simulink model "Assignment_4"  (R2023a)
settings: Solver=VariableStepAuto  StartTime=0.0  StopTime=inf  RelTol=1e-3
model workspace (MAT data in the model file):
  Initial_Weight_Vector = [0 0 0 0 0 0 0 0 0 0 0 0 0 0 0 0 0 0 0 0 0]
libraries: commchan3 x2, dspsnks4 x2, dspvision x2, dspstat3 x1
settings Model: Creator=hp  LastModifiedBy=hp

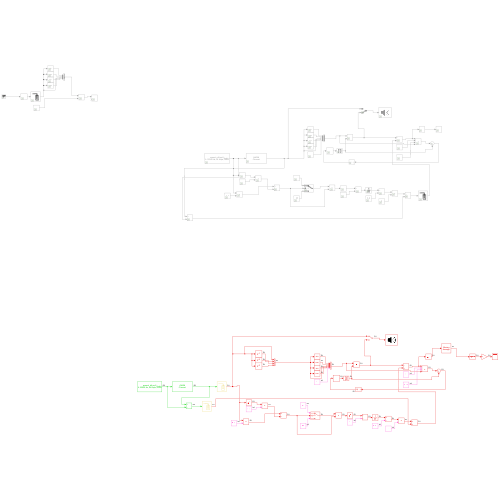
[thumbnail: Simulink's stored preview of the top-level diagram]
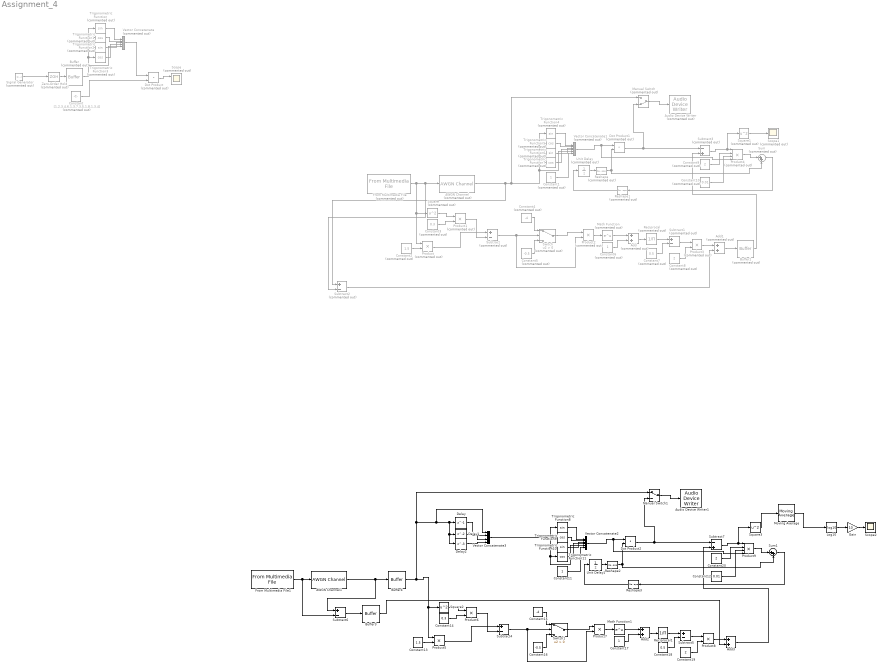
== system Assignment_4 ==
  AWGN Channel : commchan3/AWGN Channel  Commented=on  LegacyMode=off  NoiseMethod="Signal to noise ratio  (SNR)"  noiseMode="Signal to noise ratio  (SNR)"  EbNo=10  EsNo=10  SNR=10  BitsPerSymbol=1  SignalPower=1  SamplesPerSymbol=1  SymbolPeriod=1  VarianceSource=Parameter  Variance=1  RandomStream=Global stream  Seed=67  SimulateUsing=Code generation
  AWGN Channel1 : commchan3/AWGN Channel  LegacyMode=off  NoiseMethod="Signal to noise ratio  (SNR)"  noiseMode="Signal to noise ratio  (SNR)"  EbNo=10  EsNo=10  SNR=30  BitsPerSymbol=1  SignalPower=1  SamplesPerSymbol=1  SymbolPeriod=1  VarianceSource=Parameter  Variance=1  RandomStream=Global stream  Seed=67  SimulateUsing=Code generation
  Add : Sum  Commented=on
  Add1 : Sum  Commented=on
  Add2 : Sum
  Add3 : Sum
  Audio Device Writer : dspsnks4/Audio Device Writer  Commented=on  Driver=DirectSound  Device=Default  InheritSampleRate=on  SampleRate=44100  BitDepth=16-bit integer  BufferSize=4096  NumBuffers=10  DefaultOutputChannelMapping=on  OutputChannelMapping=1:2  OutputNumUnderrunSamples=off  DriverIdx=1  DeviceWarnFlag=''
  Audio Device Writer1 : dspsnks4/Audio Device Writer  Driver=DirectSound  Device=Default  InheritSampleRate=on  SampleRate=44100  BitDepth=16-bit integer  BufferSize=4096  NumBuffers=10  DefaultOutputChannelMapping=on  OutputChannelMapping=1:2  OutputNumUnderrunSamples=off  DriverIdx=1  DeviceWarnFlag=''
  Buffer : Buffer  Commented=on  N=3  V=2  OutputFrames=off
  Buffer1 : Buffer  Commented=on  N=1  OutputFrames=off
  Buffer3 : Buffer  N=1  OutputFrames=off
  Buffer4 : Buffer  N=1  OutputFrames=off
  Constant : Constant  Commented=on  Value=[1,2,3,4,6,1,3,7,3,5,1,8,1,3,4]
  Constant1 : Constant  Commented=on
  Constant10 : Constant  Commented=on  Value=0.01
  Constant11 : Constant
  Constant12 : Constant  Value=0.01
  Constant13 : Constant  Value=1.5
  Constant14 : Constant  Value=0.3
  Constant15 : Constant  Value=-4
  Constant16 : Constant  Value=-0.5
  Constant17 : Constant
  Constant18 : Constant  Value=0.5
  Constant19 : Constant  Value=2
  Constant2 : Constant  Commented=on  Value=1.5
  Constant20 : Constant  Value=2
  Constant3 : Constant  Commented=on  Value=0.3
  Constant4 : Constant  Commented=on  Value=-4
  Constant5 : Constant  Commented=on  Value=-0.5
  Constant6 : Constant  Commented=on
  Constant7 : Constant  Commented=on  Value=0.5
  Constant8 : Constant  Commented=on  Value=2
  Constant9 : Constant  Commented=on  Value=2
  Delay : Delay  DelayLength=1  InitialCondition=0
  Delay1 : Delay  InitialCondition=0
  Delay2 : Delay  DelayLength=3  InitialCondition=0
  Dot Product : DotProduct  Commented=on  OutDataTypeStr=Inherit: Inherit via internal rule
  Dot Product1 : DotProduct  Commented=on  OutDataTypeStr=Inherit: Inherit via internal rule
  Dot Product2 : DotProduct  OutDataTypeStr=Inherit: Inherit via internal rule
  From Multimedia File : dspvision/From Multimedia File  Commented=on  inputFilename=speech_dft.mp3  readRange=[1 Inf]  loop=on  numPlays=inf  outputStreams=Audio only  videoDataType=single  audioDataType=double  inheritSampleTime=on  userDefinedSampleTime=1/30  noAudioOutput=off  isIntensityVideo=off  fourcc=RGB  colorVideoFormat=Separate color signals  outputEOF=off  dataOrg=Column-major  audioFrameSize=4  computeAudioFrameSize=off  outSamplingMode=Sample based
      settings: LibrarySourceBlock=audiosources/From Multimedia File
  From Multimedia File1 : dspvision/From Multimedia File  inputFilename=speech_dft.mp3  readRange=[1 Inf]  loop=on  numPlays=inf  outputStreams=Audio only  videoDataType=single  audioDataType=double  inheritSampleTime=on  userDefinedSampleTime=1/30  noAudioOutput=off  isIntensityVideo=off  fourcc=RGB  colorVideoFormat=Separate color signals  outputEOF=off  dataOrg=Column-major  audioFrameSize=1024  computeAudioFrameSize=off  outSamplingMode=Sample based
      settings: LibrarySourceBlock=audiosources/From Multimedia File
  Gain : Gain  Gain=10
  Log10 : Math  Operator=log10
  Manual Switch : ManualSwitch  Commented=on  CurrentSetting=0
  Manual Switch1 : ManualSwitch
  Math Function : Math  Commented=on
  Math Function1 : Math
  Moving Average : dspstat3/Moving Average  Method=Sliding window  ForgettingFactorPort=off  SpecifyWindowLength=on  WindowLength=4  OverlapLength=3  AllowArbitraryInputLength=off  ForgettingFactor=0.9  SimulateUsing=Code generation
  Product{,1..3} (4 alike) : Product  Commented=on
  Product4 : Product  Commented=on  Inputs=4
  Product{5..8} (4 alike) : Product
  Product9 : Product  Inputs=4
  Reciprocal : Product  Commented=on  Inputs=/
  Reciprocal1 : Product  Inputs=/
  Reshape : Reshape  Commented=on  OutputDimensionality=Column vector (2-D)
  Reshape1 : Reshape  Commented=on
  Reshape2 : Reshape  OutputDimensionality=Column vector (2-D)
  Reshape3 : Reshape
  Scope : Scope  Commented=on  NumInputPorts=2
  Scope1 : Scope  Commented=on
  Scope2 : Scope
  Signal Generator : SignalGenerator  Commented=on  Units=rad/sec
  Square : Math  Commented=on  Operator=square
  Square1 : Math  Commented=on  Operator=square
  Square2 : Math  Operator=square
  Square3 : Math  Operator=square
  Subtract : Sum  Commented=on  Inputs=+-
  Subtract1 : Sum  Commented=on  Inputs=+-
  Subtract2 : Sum  Commented=on  Inputs=+-
  Subtract3 : Sum  Commented=on  Inputs=-+
  Subtract4 : Sum  Inputs=+-
  Subtract5 : Sum  Inputs=+-
  Subtract6 : Sum  Inputs=+-
  Subtract7 : Sum  Inputs=-+
  Sum : Sum  Commented=on  Inputs=|++
  Sum1 : Sum  Inputs=|++
  Switch : Switch  Commented=on  Criteria=u2 > Threshold  SaturateOnIntegerOverflow=off  InputSameDT=off
  Switch1 : Switch  Criteria=u2 > Threshold  SaturateOnIntegerOverflow=off  InputSameDT=off
  Trigonometric Function{,2,4,6} (4 alike) : Trigonometry  Commented=on
  Trigonometric Function{1,3,5,7} (4 alike) : Trigonometry  Commented=on  Operator=cos
  Trigonometric Function10 : Trigonometry
  Trigonometric Function11 : Trigonometry  Operator=cos
  Trigonometric Function8 : Trigonometry
  Trigonometric Function9 : Trigonometry  Operator=cos
  Unit Delay : UnitDelay  Commented=on  InitialCondition=[0 0 0 0 0 0 0 0 0 0 0 0 0 0 0 0 0 0 0 0 0]  SampleTime=-1  HasFrameUpgradeWarning=on
  Unit Delay1 : UnitDelay  InitialCondition=[0 0 0 0 0 0 0 0 0 0 0 0 0 0 0 0 0 0 0 0 0]  SampleTime=-1  HasFrameUpgradeWarning=on
  Vector Concatenate : Concatenate  Commented=on  NumInputs=5
  Vector Concatenate1 : Concatenate  Commented=on  NumInputs=6
  Vector Concatenate2 : Concatenate  NumInputs=6
  Vector Concatenate3 : Concatenate  NumInputs=4
  Zero-Order Hold : ZeroOrderHold  Commented=on  SampleTime=0.01
  wires:
  Constant/1 -> Dot Product/2
  Dot Product/1 -> Scope/1
  Signal Generator/1 -> Zero-Order Hold/1
  Zero-Order Hold/1 -> Buffer/1
  Buffer/1 -> Vector Concatenate/5, Trigonometric Function3/1, Trigonometric Function2/1, Trigonometric Function1/1, Trigonometric Function/1
  Trigonometric Function/1 -> Vector Concatenate/1
  Trigonometric Function1/1 -> Vector Concatenate/2
  Trigonometric Function2/1 -> Vector Concatenate/3
  Trigonometric Function3/1 -> Vector Concatenate/4
  Vector Concatenate/1 -> Dot Product/1
  From Multimedia File/1 -> Square/1, Product/1, Subtract2/2, AWGN Channel/1
  Trigonometric Function6/1 -> Vector Concatenate1/3
  Trigonometric Function4/1 -> Vector Concatenate1/1
  Trigonometric Function5/1 -> Vector Concatenate1/2
  Trigonometric Function7/1 -> Vector Concatenate1/4
  Constant1/1 -> Vector Concatenate1/6
  Constant2/1 -> Product/2
  Square/1 -> Product1/1
  Constant3/1 -> Product1/2
  Product/1 -> Subtract/1
  Product1/1 -> Subtract/2
  Subtract/1 -> Product2/2, Switch/2
  Constant5/1 -> Switch/3
  Constant4/1 -> Switch/1
  Switch/1 -> Product2/1
  Product2/1 -> Math Function/1
  Math Function/1 -> Add/1
  Constant6/1 -> Add/2
  Add/1 -> Reciprocal/1
  Reciprocal/1 -> Subtract1/1
  Constant7/1 -> Subtract1/2
  Subtract1/1 -> Product3/1
  Constant8/1 -> Product3/2
  Subtract2/1 -> Add1/2
  Product3/1 -> Add1/1
  Vector Concatenate1/1 -> Product4/4, Dot Product1/1
  Unit Delay/1 -> Reshape/1
  Dot Product1/1 -> Manual Switch/2, Subtract3/1
  Add1/1 -> Buffer1/1
  Subtract3/1 -> Square1/1, Product4/1
  Constant9/1 -> Product4/2
  Constant10/1 -> Product4/3
  Product4/1 -> Sum/1
  Sum/1 -> Reshape1/1
  Reshape/1 -> Dot Product1/2, Sum/2
  Reshape1/1 -> Unit Delay/1
  Manual Switch/1 -> Audio Device Writer/1
  AWGN Channel/1 -> Manual Switch/1, Vector Concatenate1/5, Trigonometric Function7/1, Trigonometric Function6/1, Trigonometric Function5/1, Trigonometric Function4/1, Subtract2/1
  Buffer1/1 -> Subtract3/2
  Square1/1 -> Scope1/1
  Constant12/1 -> Product9/3
  Constant20/1 -> Product9/2
  Manual Switch1/1 -> Audio Device Writer1/1
  Constant13/1 -> Product5/2
  Sum1/1 -> Reshape3/1
  Reshape3/1 -> Unit Delay1/1
  Add3/1 -> Subtract7/2
  Constant19/1 -> Product8/2
  Product9/1 -> Sum1/1
  Math Function1/1 -> Add2/1
  Unit Delay1/1 -> Reshape2/1
  Subtract4/1 -> Product7/2, Switch1/2
  Constant18/1 -> Subtract5/2
  Constant11/1 -> Vector Concatenate2/6
  Constant15/1 -> Switch1/1
  Add2/1 -> Reciprocal1/1
  Product5/1 -> Subtract4/1
  Switch1/1 -> Product7/1
  Trigonometric Function11/1 -> Vector Concatenate2/4
  Trigonometric Function9/1 -> Vector Concatenate2/2
  Trigonometric Function10/1 -> Vector Concatenate2/3
  Trigonometric Function8/1 -> Vector Concatenate2/1
  Constant17/1 -> Add2/2
  Product6/1 -> Subtract4/2
  Subtract5/1 -> Product8/1
  Product8/1 -> Add3/1
  Square2/1 -> Product6/1
  AWGN Channel1/1 -> Buffer4/1, Subtract6/1
  Square3/1 -> Moving Average/1
  Constant16/1 -> Switch1/3
  Subtract7/1 -> Square3/1, Product9/1
  Constant14/1 -> Product6/2
  Vector Concatenate2/1 -> Product9/4, Dot Product2/1
  Reciprocal1/1 -> Subtract5/1
  Product7/1 -> Math Function1/1
  Reshape2/1 -> Dot Product2/2, Sum1/2
  Dot Product2/1 -> Manual Switch1/2, Subtract7/1
  Vector Concatenate3/1 -> Vector Concatenate2/5, Trigonometric Function11/1, Trigonometric Function10/1, Trigonometric Function9/1, Trigonometric Function8/1
  From Multimedia File1/1 -> Subtract6/2, AWGN Channel1/1
  Subtract6/1 -> Buffer3/1
  Log10/1 -> Gain/1
  Gain/1 -> Scope2/1
  Buffer3/1 -> Add3/2
  Buffer4/1 -> Vector Concatenate3/1, Delay2/1, Delay1/1, Delay/1, Manual Switch1/1, Square2/1, Product5/1
  Delay2/1 -> Vector Concatenate3/4
  Delay1/1 -> Vector Concatenate3/3
  Delay/1 -> Vector Concatenate3/2
  Moving Average/1 -> Log10/1
